simulink model "euler321_12B"  (R2022a)
settings: Solver=ode3  StartTime=0.0  StopTime=10  FixedStep=0.01  RelTol=1e-3  EnableMultiTasking=on
values from neighbouring files (symbols this model uses):
  toll = 0.01    [SettingEU.m]
undefined symbols (not defined in the file or in its folder): Hecate_phiRamp, Hecate_psiDelay, Hecate_thetaFreq, Hecate_VectX, Hecate_VectY, Hecate_VectZ
libraries: sharedutil x4
settings Model: Creator=elliocm  LastModifiedBy=fedformi_new
settings SolverCC: AlgebraicLoopSolver=TrustRegion
settings DataIOCC: SaveFormat=StructureWithTime  SignalLoggingSaveFormat=ModelDataLogs
settings OptimizationCC: ExpressionDepthLimit=2147483647  LifeSpan=inf
settings DebuggingCC: UnderspecifiedInitializationDetection=Classic  MergeDetectMultiDrivingBlocksExec=none  SolverPrmCheckMsg=warning  FcnCallInpInsideContextMsg=warning  UnconnectedInputMsg=warning  UnconnectedOutputMsg=warning  UnconnectedLineMsg=warning  StateNameClashWarn=warning  SFUnexpectedBacktrackingDiag=warning  SFNoUnconditionalDefaultTransitionDiag=warning  SFExecutionAtInitializationDiag=none  SFMachineParentedDataDiag=warning  ArithmeticOperatorsInVariantConditions=warning
settings HardwareCC: ProdBitPerPointer=32  ProdBitPerSizeT=32  ProdBitPerPtrDiffT=32  ProdLargestAtomicFloat=None  ProdIntDivRoundTo=Undefined  ProdEndianess=Unspecified  ProdWordSize=32  ProdHWDeviceType=32-bit Generic
settings ModelReferenceCC: PropagateSignalLabelsOutOfModel=off
settings SFSimCC: SimUseLocalCustomCode=off  CustomCodeUndefinedFunction=UseInterfaceOnly
settings RTWCC: RTWUseLocalCustomCode=off
settings CodeAppCC: StateflowObjectComments=on
settings GRTTargetCC: TargetLangStandard=C89/C90 (ANSI)  CombineOutputUpdateFcns=off  GRTInterface=on
settings ConfigComp: CovMetricSettings=dw  CovSaveCumulativeToWorkspaceVar=on  CovSaveSingleToWorkspaceVar=on  CovExternalEMLEnable=off

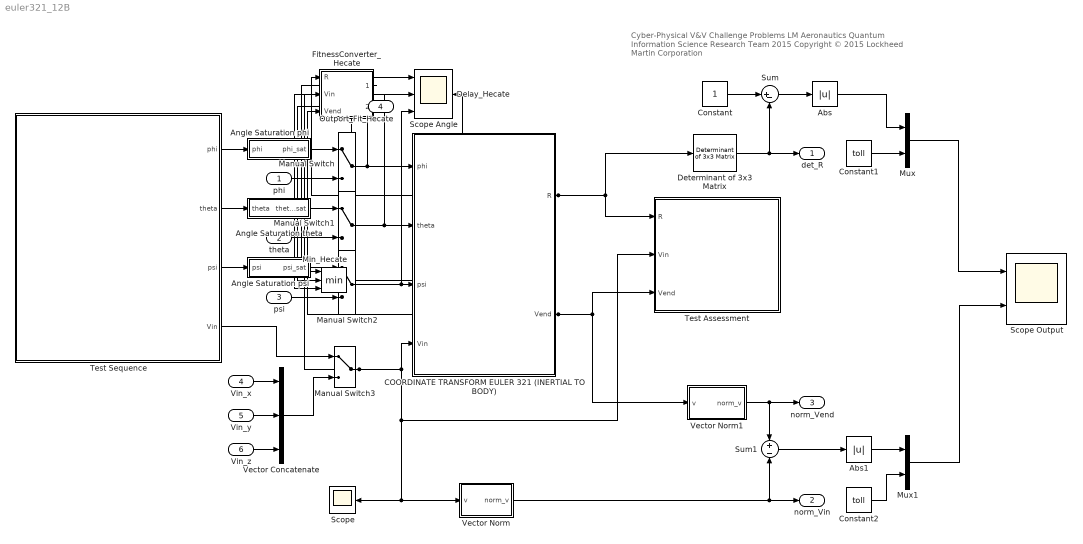
== system euler321_12B ==
  note: Cyber-Physical V&V Challenge Problems
      | LM Aeronautics Quantum Information Science Research Team 2015
      | Copyright © 2015 Lockheed Martin Corporation
  phi : Inport  OutDataTypeStr=double
  theta : Inport  Port=2  OutDataTypeStr=double
  psi : Inport  Port=3  OutDataTypeStr=double
  Vin_x : Inport  Port=4  OutDataTypeStr=double
  Vin_y : Inport  Port=5  OutDataTypeStr=double
  Vin_z : Inport  Port=6  OutDataTypeStr=double
  Abs : Abs  SaturateOnIntegerOverflow=off
  Abs1 : Abs  SaturateOnIntegerOverflow=off
  Angle Saturation phi : Subsystem
  Angle Saturation psi : Subsystem
  Angle Saturation theta : Subsystem
  COORDINATE TRANSFORM EULER 321 (INERTIAL TO BODY) : Subsystem
  Constant : Constant
  Constant1 : Constant  Value=toll
  Constant2 : Constant  Value=toll
  Delay_Hecate : Delay  DelayLength=1  InitialCondition=Inf
  Determinant of 3x3 Matrix : sharedutil/Determinant of 3x3 Matrix  aMode=aMode
      settings: SourceProductBaseCode=AE,PW,DR,MT,VE
  FitnessConverter_Hecate : Stateflow chart  TreatAsAtomicUnit=on
  Manual Switch{,1..3} (4 alike) : ManualSwitch
  Min_Hecate : MinMax  Inputs=3
  Mux : Mux  Inputs=2
  Mux1 : Mux  Inputs=2
  Scope : Scope
  Scope Angle : Scope  NumInputPorts=3
  Scope Output : Scope  NumInputPorts=2
  Sum : Sum  Inputs=|+-
  Sum1 : Sum  Inputs=+-
  Test Assessment : Test Sequence  TreatAsAtomicUnit=on
  Test Sequence : Test Sequence  TreatAsAtomicUnit=on
  Vector Concatenate : Concatenate  NumInputs=3
  Vector Norm : Subsystem
  Vector Norm1 : Subsystem
  det_R : Outport
  norm_Vin : Outport  Port=2
  norm_Vend : Outport  Port=3
  Outport_Fit_Hecate : Outport  Port=4
  wires:
  COORDINATE TRANSFORM EULER 321 (INERTIAL TO BODY)/1(R) -> Test Assessment/1(R), Determinant of 3x3 Matrix/1, FitnessConverter_Hecate/1(R)
  COORDINATE TRANSFORM EULER 321 (INERTIAL TO BODY)/2(Vend) -> Vector Norm1/1(v), Test Assessment/3(Vend), FitnessConverter_Hecate/3(Vend)
  Manual Switch/1 -> COORDINATE TRANSFORM EULER 321 (INERTIAL TO BODY)/1(phi), Scope Angle/1
  Manual Switch1/1 -> COORDINATE TRANSFORM EULER 321 (INERTIAL TO BODY)/2(theta), Scope Angle/2
  Manual Switch2/1 -> Scope Angle/3, COORDINATE TRANSFORM EULER 321 (INERTIAL TO BODY)/3(psi)
  Manual Switch3/1 -> Vector Norm/1(v), Scope/1, Test Assessment/2(Vin), COORDINATE TRANSFORM EULER 321 (INERTIAL TO BODY)/4(Vin), FitnessConverter_Hecate/2(Vin)
  phi/1 -> Manual Switch/2
  Test Sequence/1(phi) -> Angle Saturation phi/1(phi)
  theta/1 -> Manual Switch1/2
  Test Sequence/2(theta) -> Angle Saturation theta/1(theta)
  psi/1 -> Manual Switch2/2
  Test Sequence/3(psi) -> Angle Saturation psi/1(psi)
  Test Sequence/4(Vin) -> Manual Switch3/1
  Vin_x/1 -> Vector Concatenate/1
  Vin_y/1 -> Vector Concatenate/2
  Vin_z/1 -> Vector Concatenate/3
  Vector Concatenate/1 -> Manual Switch3/2
  Determinant of 3x3 Matrix/1 -> det_R/1, Sum/2
  Vector Norm/1(norm_v) -> Sum1/2, norm_Vin/1
  Vector Norm1/1(norm_v) -> Sum1/1, norm_Vend/1
  Angle Saturation phi/1(phi_sat) -> Manual Switch/1
  Angle Saturation psi/1(psi_sat) -> Manual Switch2/1
  Angle Saturation theta/1(theta_sat) -> Manual Switch1/1
  Constant/1 -> Sum/1
  Sum/1 -> Abs/1
  Abs/1 -> Mux/1
  Mux/1 -> Scope Output/1
  Constant1/1 -> Mux/2
  Constant2/1 -> Mux1/2
  Abs1/1 -> Mux1/1
  Sum1/1 -> Abs1/1
  Mux1/1 -> Scope Output/2
  FitnessConverter_Hecate/1(fitness_1) -> Min_Hecate/1
  FitnessConverter_Hecate/2(fitness_2) -> Min_Hecate/2
  Min_Hecate/1 -> Delay_Hecate/1, Outport_Fit_Hecate/1
  Delay_Hecate/1 -> Min_Hecate/3

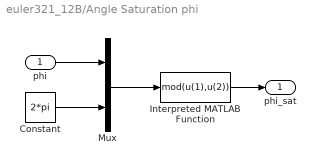
== system euler321_12B/Angle Saturation phi ==
  phi : Inport
  Constant : Constant  Value=2*pi
  Interpreted MATLAB Function : MATLABFcn  MATLABFcn=mod(u(1),u(2))
  Mux : Mux  Inputs=2
  phi_sat : Outport
  wires:
  phi/1 -> Mux/1
  Interpreted MATLAB Function/1 -> phi_sat/1
  Constant/1 -> Mux/2
  Mux/1 -> Interpreted MATLAB Function/1

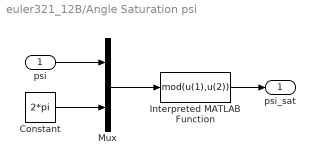
== system euler321_12B/Angle Saturation psi ==
  psi : Inport
  Constant : Constant  Value=2*pi
  Interpreted MATLAB Function : MATLABFcn  MATLABFcn=mod(u(1),u(2))
  Mux : Mux  Inputs=2
  psi_sat : Outport
  wires:
  psi/1 -> Mux/1
  Interpreted MATLAB Function/1 -> psi_sat/1
  Constant/1 -> Mux/2
  Mux/1 -> Interpreted MATLAB Function/1

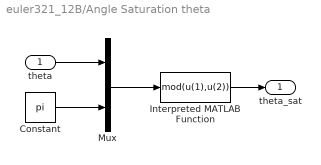
== system euler321_12B/Angle Saturation theta ==
  theta : Inport
  Constant : Constant  Value=pi
  Interpreted MATLAB Function : MATLABFcn  MATLABFcn=mod(u(1),u(2))
  Mux : Mux  Inputs=2
  theta_sat : Outport
  wires:
  theta/1 -> Mux/1
  Interpreted MATLAB Function/1 -> theta_sat/1
  Constant/1 -> Mux/2
  Mux/1 -> Interpreted MATLAB Function/1

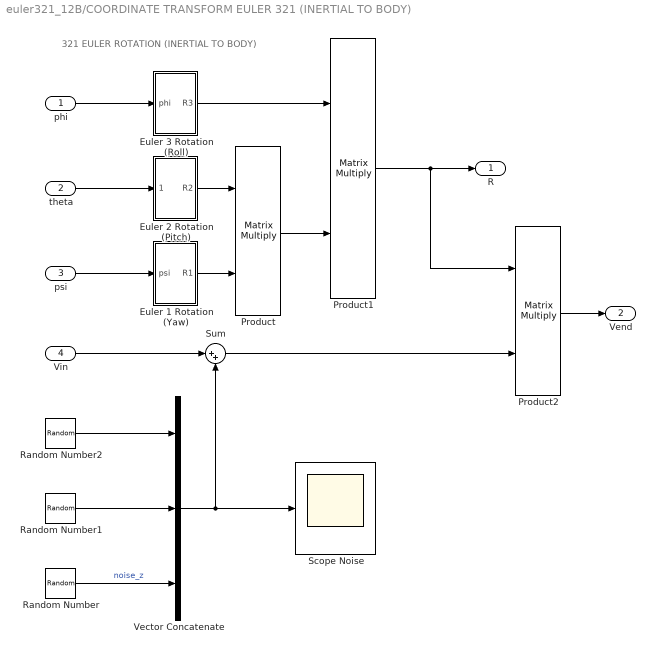
== system euler321_12B/COORDINATE TRANSFORM EULER 321 (INERTIAL TO BODY) ==
  note: 321 EULER ROTATION (INERTIAL TO BODY)
  phi : Inport
  theta : Inport  Port=2
  psi : Inport  Port=3
  Vin : Inport  Port=4
  Euler 1 Rotation (Yaw) : Subsystem
  Euler 2 Rotation (Pitch) : Subsystem
  Euler 3 Rotation (Roll) : Subsystem
  Product : Product  Multiplication=Matrix(*)  RndMeth=Zero
  Product1 : Product  Multiplication=Matrix(*)  RndMeth=Zero
  Product2 : Product  Multiplication=Matrix(*)  RndMeth=Zero
  Random Number : RandomNumber  Variance=1e-5  Seed=2  SampleTime=0.01
  Random Number1 : RandomNumber  Variance=1e-6  Seed=1  SampleTime=0.01
  Random Number2 : RandomNumber  Variance=1e-6  SampleTime=0.01
  Scope Noise : Scope
  Sum : Sum  Inputs=|++
  Vector Concatenate : Concatenate  NumInputs=3
  R : Outport
  Vend : Outport  Port=2
  wires:
  Euler 2 Rotation (Pitch)/1(R2) -> Product/1
  Euler 1 Rotation (Yaw)/1(R1) -> Product/2
  Euler 3 Rotation (Roll)/1(R3) -> Product1/1
  Product/1 -> Product1/2
  Product1/1 -> R/1, Product2/1
  Product2/1 -> Vend/1
  phi/1 -> Euler 3 Rotation (Roll)/1(phi)
  theta/1 -> Euler 2 Rotation (Pitch)/1(theta)
  psi/1 -> Euler 1 Rotation (Yaw)/1(psi)
  Vin/1 -> Sum/1
  Sum/1 -> Product2/2
  Vector Concatenate/1 -> Scope Noise/1, Sum/2
  Random Number2/1 -> Vector Concatenate/1
  Random Number1/1 -> Vector Concatenate/2
  Random Number/1 -> Vector Concatenate/3  "noise_z"

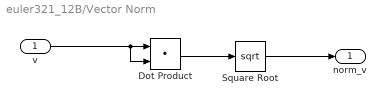
== system euler321_12B/Vector Norm ==
  v : Inport
  Dot Product : DotProduct  OutMin=0  OutDataTypeStr=Inherit: Inherit via internal rule
  Square Root : Sqrt
  norm_v : Outport
  wires:
  Square Root/1 -> norm_v/1
  Dot Product/1 -> Square Root/1
  v/1 -> Dot Product/2, Dot Product/1

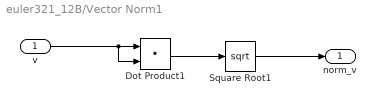
== system euler321_12B/Vector Norm1 ==
  v : Inport
  Dot Product1 : DotProduct  OutMin=0  OutDataTypeStr=Inherit: Inherit via internal rule
  Square Root1 : Sqrt
  norm_v : Outport
  wires:
  Square Root1/1 -> norm_v/1
  v/1 -> Dot Product1/1, Dot Product1/2
  Dot Product1/1 -> Square Root1/1

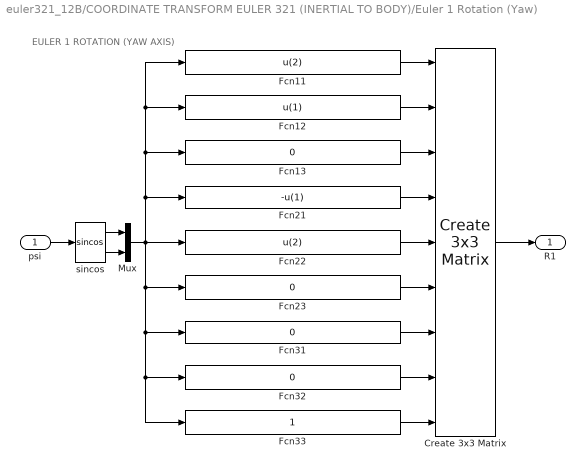
== system euler321_12B/COORDINATE TRANSFORM EULER 321 (INERTIAL TO BODY)/Euler 1 Rotation (Yaw) ==
  note: EULER 1 ROTATION (YAW AXIS)
  psi : Inport
  Create 3x3 Matrix : sharedutil/Create 3x3 Matrix  aMode=aMode
  Fcn11 : Fcn  Expr=u(2)
  Fcn12 : Fcn  Expr=u(1)
  Fcn{13,23,31..32} (4 alike) : Fcn  Expr=0
  Fcn21 : Fcn  Expr=-u(1)
  Fcn22 : Fcn  Expr=u(2)
  Fcn33 : Fcn  Expr=1
  Mux : Mux  Inputs=2
  sincos : Trigonometry  Operator=sincos
  R1 : Outport  PortDimensions=[3,3]
  wires:
  psi/1 -> sincos/1
  Create 3x3 Matrix/1 -> R1/1
  sincos/1 -> Mux/1
  sincos/2 -> Mux/2
  Mux/1 -> Fcn32/1, Fcn33/1, Fcn31/1, Fcn23/1, Fcn22/1, Fcn11/1, Fcn12/1, Fcn13/1, Fcn21/1
  Fcn11/1 -> Create 3x3 Matrix/1
  Fcn12/1 -> Create 3x3 Matrix/2
  Fcn13/1 -> Create 3x3 Matrix/3
  Fcn21/1 -> Create 3x3 Matrix/4
  Fcn31/1 -> Create 3x3 Matrix/7
  Fcn22/1 -> Create 3x3 Matrix/5
  Fcn23/1 -> Create 3x3 Matrix/6
  Fcn32/1 -> Create 3x3 Matrix/8
  Fcn33/1 -> Create 3x3 Matrix/9

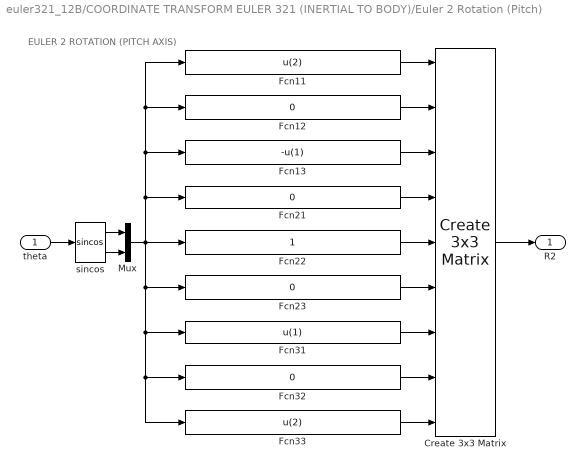
== system euler321_12B/COORDINATE TRANSFORM EULER 321 (INERTIAL TO BODY)/Euler 2 Rotation (Pitch) ==
  note: EULER 2 ROTATION (PITCH AXIS)
  theta : Inport
  Create 3x3 Matrix : sharedutil/Create 3x3 Matrix  aMode=aMode
  Fcn11 : Fcn  Expr=u(2)
  Fcn{12,21,23,32} (4 alike) : Fcn  Expr=0
  Fcn13 : Fcn  Expr=-u(1)
  Fcn22 : Fcn  Expr=1
  Fcn31 : Fcn  Expr=u(1)
  Fcn33 : Fcn  Expr=u(2)
  Mux : Mux  Inputs=2
  sincos : Trigonometry  Operator=sincos
  R2 : Outport  PortDimensions=[3,3]
  wires:
  theta/1 -> sincos/1
  Create 3x3 Matrix/1 -> R2/1
  sincos/1 -> Mux/1
  sincos/2 -> Mux/2
  Mux/1 -> Fcn32/1, Fcn33/1, Fcn31/1, Fcn23/1, Fcn22/1, Fcn11/1, Fcn12/1, Fcn13/1, Fcn21/1
  Fcn11/1 -> Create 3x3 Matrix/1
  Fcn12/1 -> Create 3x3 Matrix/2
  Fcn13/1 -> Create 3x3 Matrix/3
  Fcn21/1 -> Create 3x3 Matrix/4
  Fcn31/1 -> Create 3x3 Matrix/7
  Fcn22/1 -> Create 3x3 Matrix/5
  Fcn23/1 -> Create 3x3 Matrix/6
  Fcn32/1 -> Create 3x3 Matrix/8
  Fcn33/1 -> Create 3x3 Matrix/9

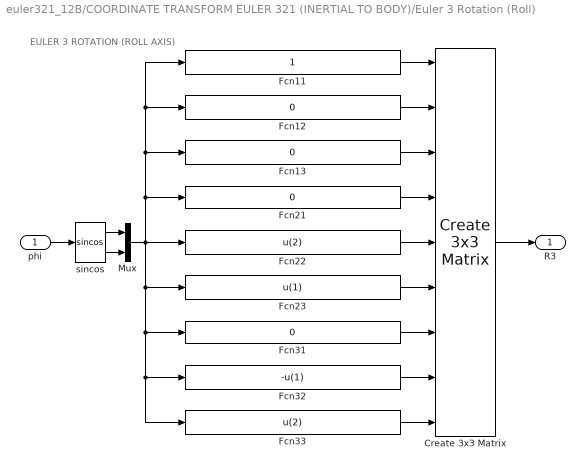
== system euler321_12B/COORDINATE TRANSFORM EULER 321 (INERTIAL TO BODY)/Euler 3 Rotation (Roll) ==
  note: EULER 3 ROTATION (ROLL AXIS)
  phi : Inport
  Create 3x3 Matrix : sharedutil/Create 3x3 Matrix  aMode=aMode
  Fcn11 : Fcn  Expr=1
  Fcn{12..13,21,31} (4 alike) : Fcn  Expr=0
  Fcn22 : Fcn  Expr=u(2)
  Fcn23 : Fcn  Expr=u(1)
  Fcn32 : Fcn  Expr=-u(1)
  Fcn33 : Fcn  Expr=u(2)
  Mux : Mux  Inputs=2
  sincos : Trigonometry  Operator=sincos
  R3 : Outport  PortDimensions=[3,3]
  wires:
  phi/1 -> sincos/1
  Create 3x3 Matrix/1 -> R3/1
  sincos/1 -> Mux/1
  sincos/2 -> Mux/2
  Mux/1 -> Fcn32/1, Fcn33/1, Fcn31/1, Fcn23/1, Fcn22/1, Fcn11/1, Fcn12/1, Fcn13/1, Fcn21/1
  Fcn11/1 -> Create 3x3 Matrix/1
  Fcn12/1 -> Create 3x3 Matrix/2
  Fcn13/1 -> Create 3x3 Matrix/3
  Fcn21/1 -> Create 3x3 Matrix/4
  Fcn31/1 -> Create 3x3 Matrix/7
  Fcn22/1 -> Create 3x3 Matrix/5
  Fcn23/1 -> Create 3x3 Matrix/6
  Fcn32/1 -> Create 3x3 Matrix/8
  Fcn33/1 -> Create 3x3 Matrix/9

== stateflow chart euler321_12B/Test Assessment ==
  state step_1
    verify(abs(norm(Vin)-norm(Vend)) <= toll)
    verify(det(R) <= 1+toll && det(R) >= 1-toll)
  (default) -> step_1
  data: R input; Vin input; Vend input; toll parameter

== stateflow chart euler321_12B/FitnessConverter_Hecate ==
  state step_1
    fitness_1 = toll-(abs(norm(Vin)-norm(Vend)));
    fitness_2 = min([1+toll-(det(R));det(R)-(1-toll);]);
  (default) -> step_1
  data: R input; Vin input; Vend input; toll parameter; fitness_1 output; fitness_2 output

== stateflow chart euler321_12B/Test Sequence ==
  state step_1
    phi = pi*ramp(t*Hecate_phiRamp);
    theta = pi/2+pi/2*sin(t*Hecate_thetaFreq);
    psi = -pi/3+pi*heaviside(t-Hecate_psiDelay);
    Vin = [Hecate_VectX; Hecate_VectY; Hecate_VectZ];
    settings: description=|
        | phi and psi are between 0 and 2*pi.
        | theta is between 0 and pi.
  (default) -> step_1
  data: phi output; theta output; psi output; Vin output; Hecate_VectX parameter; Hecate_phiRamp parameter; Hecate_thetaFreq parameter; Hecate_psiDelay parameter; Hecate_VectY parameter; Hecate_VectZ parameter
